simulink model "SIM_Patria_Microgrid"  (R2020b)
settings: Solver=ode23tb  StartTime=0.0  StopTime=24*60*60  FixedStep=1/(1000)  MaxStep=60  RelTol=1e-4
PreLoadFcn:
  | run('sim_initial_values.m')
StartFcn:
  | open_system('SIM_Patria_Microgrid/Scopes/ScopeSPS')
values from neighbouring files (symbols this model uses):
  data = get_scenario(1)    [sim_initial_values.m]
undefined symbols (not defined in the file or in its folder): Angle, Magnitude, params
libraries: powerlib x34, simulink x4
settings Model: ModifiedByFormat=SPS  ExtModeTrigMode=oneshot  ExtModeArmWhenConnect=off  Creator=MathWorks  LastModifiedBy=SPS
settings SolverCC: InitialStep=1e-4  ZeroCrossAlgorithm=Adaptive
settings DataIOCC: SaveFormat=Array  SignalLoggingSaveFormat=ModelDataLogs  SaveOutput=off  SaveTime=off  ReturnWorkspaceOutputs=off  SignalLoggingName=sigsOut
settings OptimizationCC: BooleanDataType=off  ExpressionDepthLimit=2147483647  InitFltsAndDblsToZero=on  LifeSpan=inf
settings DebuggingCC: AlgebraicLoopMsg=none  SaveWithParameterizedLinksMsg=none  UnderspecifiedInitializationDetection=Classic  MergeDetectMultiDrivingBlocksExec=none  SignalResolutionControl=TryResolveAllWithWarning  MultiTaskDSMMsg=warning  MultiTaskCondExecSysMsg=none  FcnCallInpInsideContextMsg=warning  AllowSymbolicDim=off  StateNameClashWarn=warning  SFUnexpectedBacktrackingDiag=warning  SFNoUnconditionalDefaultTransitionDiag=warning  SFExecutionAtInitializationDiag=none  ArithmeticOperatorsInVariantConditions=warning
settings HardwareCC: ProdBitPerPointer=32  ProdBitPerSizeT=32  ProdBitPerPtrDiffT=32  ProdLargestAtomicFloat=None  ProdIntDivRoundTo=Undefined  ProdEndianess=Unspecified  ProdWordSize=32  ProdHWDeviceType=32-bit Generic  TargetUnknown=on
settings ModelReferenceCC: PropagateSignalLabelsOutOfModel=off
settings SFSimCC: SimUseLocalCustomCode=off  CustomCodeUndefinedFunction=UseInterfaceOnly
settings RTWCC: RTWUseLocalCustomCode=off
settings CodeAppCC: StateflowObjectComments=on
settings GRTTargetCC: TargetFcnLib=ansi_tfl_tmw.mat  TargetLangStandard=C89/C90 (ANSI)  CombineOutputUpdateFcns=off  GRTInterface=on
settings ConfigComp: CovMetricSettings=dw  CovSaveCumulativeToWorkspaceVar=on  CovSaveSingleToWorkspaceVar=on  CovExternalEMLEnable=off  CovSFcnEnable=off
settings SimscapeCC: SimscapeNormalizeSystem=off

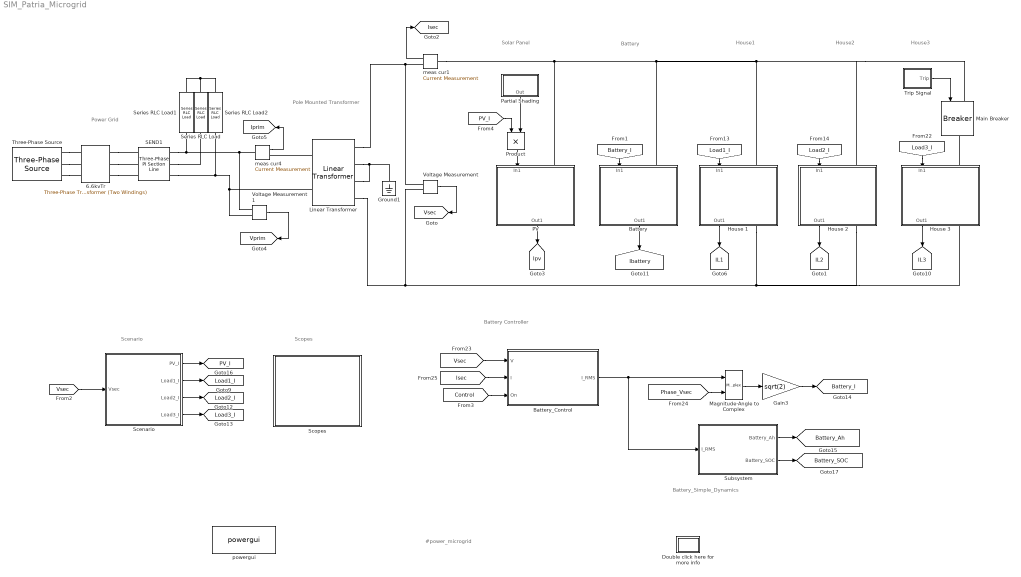
== system SIM_Patria_Microgrid ==
  note: Power Grid
  note: Pole Mounted
      | Transformer
  note: Solar Panel
  note: Battery
  note: House1
  note: House2
  note: House3
  note: Battery_Simple_Dynamics
  note: Battery Controller
  note: Scenario
  note: Scopes
  note: #power_microgrid
  6.6kvTr : powerlib/Elements/Three-Phase Transformer (Two Windings)  Winding1Connection=Yg  Winding2Connection=Y  CoreType=Three single-phase transformers  SetSaturation=off  Hysteresis=off  DataFile='hysteresis'  SetInitialFlux=off  Measurements=None  UNITS=pu  NominalPower=[ 10e6 , 60 ]  Winding1=[ 66e3 , 0.002 , 0.08 ]  Winding2=[6.6e3 , 0.002 , 0.08 ]  Rm=500  Lm=500  L0=0.5  Saturation=[ 0,0 ; 0.0024,1.2 ; 1.0,1.52 ]  InitialFluxes=[ 0.8 , -0.8 , 0.7 ]  BreakLoop=on  DiscreteSolver=Trapezoidal iterative  DataType=off  TransfoNumber=1
  Battery : Subsystem
      mask Display: image(imread(fullfile(matlabroot,'toolbox/physmod/powersys/DR/DRdemo/Battery.jpg')))
  Battery_Control : Subsystem
  Double click here for more info : Subsystem
      settings: OpenFcn=showdemo(bdroot(gcb))
      mask Display: disp('?')
  Gain3 : Gain  Gain=sqrt(2)
  Ground1 : powerlib/Elements/Ground  LConnTagsString=a
  House 1 : Subsystem
      mask Display: image(imread('house.jpg'))
  House 2 : Subsystem
      mask Display: image(imread('house.jpg'))
  House 3 : Subsystem
      mask Display: image(imread('house.jpg'))
  Linear Transformer : powerlib/Elements/Linear Transformer  UNITS=pu  NominalPower=[75e3 60]  winding1=[ 6600 0.00005 0.0002 ]  winding2=[ 100 0.00005 0.0002 ]  ThreeWindings=on  winding3=[ 100 0.00005 0.0002 ]  RmLm=[ 50 50 ]  Measurements=None  DataType=off
  Magnitude-Angle to Complex : MagnitudeAngleToComplex
  Main Breaker : powerlib/Elements/Breaker  InitialState=1  SwitchingTimes=[0 10 ]+8*3600  External=on  BreakerResistance=0.001  SnubberResistance=1e6  SnubberCapacitance=inf  Measurements=None  MoreParameters=off  NoBreakLoop=off
  PV : Subsystem
      mask Display: image(imread('pv.jpg'))
  Partial Shading : Subsystem  mask(Signal Disturbance){Hour=11, Minute=0, Second=0, Duration=20, Factor=0.3}
      mask prompts: Duration "Duration (s):"
      mask help: Within the specified time range defined by Start and Duration parameters, output is set to 'Factor'. Outside the specified time range output is kept at 1.0.
      mask init:
      | T2=(Hour-1)*60*60;    % Hour in seconds
      | T3=(Minute-1)*60;  % Minute in seconds
      | Ton=T2+T3+(Second-1);    % Beginning of fault (s)
      | Toff=Ton+Duration; % End of fault (s)
      mask TypeOptions Hour: 0 |      1 |      2 |      3 |      4 |      5 |      6 |      7 |      8 |      9 |     10 |     11 |     12 |     13 |     14 |     15 |     16 |     17 |     18 |     19 |     20 |     21 |     22 |     23
      mask TypeOptions Minute: 0 |      1 |      2 |      3 |      4 |      5 |      6 |      7 |      8 |      9 |     10 |     11 |     12 |     13 |     14 |     15 |     16 |     17 |     18 |     19 |     20 |     21 |     22 |     23 |     24 |     25 |     26 |     27 |     28 |     29 |     30 |     31 |     32 |     33 |     34 |     35 |     36 |     37 |     38 |     39 |     40 |     41 |     42 |     43 |     44 |     45 |     46 |     47 |     48 |     49 |     50 |     51 |     52 |     53 |     54 |     55 |     56 |     57 |     58 |     59
      mask TypeOptions Second: 0 |      1 |      2 |      3 |      4 |      5 |      6 |      7 |      8 |      9 |     10 |     11 |     12 |     13 |     14 |     15 |     16 |     17 |     18 |     19 |     20 |     21 |     22 |     23 |     24 |     25 |     26 |     27 |     28 |     29 |     30 |     31 |     32 |     33 |     34 |     35 |     36 |     37 |     38 |     39 |     40 |     41 |     42 |     43 |     44 |     45 |     46 |     47 |     48 |     49 |     50 |     51 |     52 |     53 |     54 |     55 |     56 |     57 |     58 |     59
      mask DialogControl Control2 Prompt: Start:
  Product : Product
  SEND1 : powerlib/Elements/Three-Phase PI Section Line  LConnTagsString=a|b|c  RConnTagsString=A|B|C  Length=1  Frequency=50  Resistances=[ 0.01273 0.3864]  Inductances="[ 0.9337e-3  4.1264e-3]"  Capacitances=[12.74e-9 7.751e-9]
  Scenario : Subsystem
  Scopes : Subsystem
  Series RLC Load : powerlib/Elements/Series RLC Load  LConnTagsString=a  RConnTagsString=__new0  NominalVoltage=1000  NominalFrequency=50  ActivePower=10e3  InductivePower=100  CapacitivePower=100  Setx0=off  InitialVoltage=0  SetiL0=off  InitialCurrent=0  Measurements=None  LoadType=constant Z
  Series RLC Load1 : powerlib/Elements/Series RLC Load  LConnTagsString=a  RConnTagsString=__new0  NominalVoltage=1000  NominalFrequency=50  ActivePower=100e3  InductivePower=100  CapacitivePower=100  Setx0=off  InitialVoltage=0  SetiL0=off  InitialCurrent=0  Measurements=None  LoadType=constant Z
  Series RLC Load2 : powerlib/Elements/Series RLC Load  LConnTagsString=a  RConnTagsString=__new0  NominalVoltage=1000  NominalFrequency=50  ActivePower=10e3  InductivePower=100  CapacitivePower=100  Setx0=off  InitialVoltage=0  SetiL0=off  InitialCurrent=0  Measurements=None  LoadType=constant Z
  Subsystem : Subsystem  mask{AH=5000}
      mask prompts: AH "Capacity[Ah]"
      mask Display: image(imread(fullfile(matlabroot,'toolbox/physmod/powersys/DR/DRdemo/Battery.jpg')))
  Three-Phase Source : powerlib/Electrical Sources/Three-Phase Source  InternalConnection=Yg  VoltagePhases=off  Voltage=66e3  PhaseAngle=0  Voltage_phases=[25e3 25e3 25e3]/sqrt(3)  PhaseAngles_phases=[0 -120 +120]  Frequency=params.network.frequency  NonIdealSource=on  SpecifyImpedance=on  Resistance=0.8929  Inductance=16.58e-3  ShortCircuitLevel=100e6  BaseVoltage=25e3  XRratio=7  BusType=swing  Pref=0  Qref=0  Prefabc=[10e3, 10e3, 10e3]  Qrefabc=[0, 0, 0]  Qmin=-inf  Qmax=inf
  Trip Signal : Subsystem  mask(Trip Signal for House Main Breaker){Hour=8, Minute=0, Second=0, FaultDuration=0}
      mask prompts: FaultDuration "Fault duration (s):"
      mask init:
      | T2=(Hour-1)*60*60;    % Hour in seconds
      | T3=(Minute-1)*60;  % Minute in seconds
      | Ton=T2+T3+(Second-1);    % Beginning of fault (s)
      | Toff=Ton+FaultDuration; % End of fault (s)
      mask TypeOptions Hour: 0 |      1 |      2 |      3 |      4 |      5 |      6 |      7 |      8 |      9 |     10 |     11 |     12 |     13 |     14 |     15 |     16 |     17 |     18 |     19 |     20 |     21 |     22 |     23
      mask TypeOptions Minute: 0 |      1 |      2 |      3 |      4 |      5 |      6 |      7 |      8 |      9 |     10 |     11 |     12 |     13 |     14 |     15 |     16 |     17 |     18 |     19 |     20 |     21 |     22 |     23 |     24 |     25 |     26 |     27 |     28 |     29 |     30 |     31 |     32 |     33 |     34 |     35 |     36 |     37 |     38 |     39 |     40 |     41 |     42 |     43 |     44 |     45 |     46 |     47 |     48 |     49 |     50 |     51 |     52 |     53 |     54 |     55 |     56 |     57 |     58 |     59
      mask TypeOptions Second: 0 |      1 |      2 |      3 |      4 |      5 |      6 |      7 |      8 |      9 |     10 |     11 |     12 |     13 |     14 |     15 |     16 |     17 |     18 |     19 |     20 |     21 |     22 |     23 |     24 |     25 |     26 |     27 |     28 |     29 |     30 |     31 |     32 |     33 |     34 |     35 |     36 |     37 |     38 |     39 |     40 |     41 |     42 |     43 |     44 |     45 |     46 |     47 |     48 |     49 |     50 |     51 |     52 |     53 |     54 |     55 |     56 |     57 |     58 |     59
      mask DialogControl Control2 Prompt: Fault timing:
  Voltage Measurement : powerlib/Measurements/Voltage Measurement  PhasorSimulation=on  OutputType=Complex  PSBequivalent=0
  Voltage Measurement1 : powerlib/Measurements/Voltage Measurement  PhasorSimulation=on  OutputType=Magnitude-Angle  PSBequivalent=0
  meas cur1 : powerlib/Measurements/Current Measurement  PhasorSimulation=on  OutputType=Complex  PSBequivalent=0
  meas cur4 : powerlib/Measurements/Current Measurement  PhasorSimulation=on  OutputType=Magnitude-Angle  PSBequivalent=0
  powergui : powerlib/powergui  SimulationMode=Phasor  SampleTime=1/60/100  frequency=50  Iterations=50  frequencyindice=60  Pbase=100e6  ErrMax=1e-4  UnitsV=kV  UnitsW=MW  buscounter=0  FunctionMessages=off  echomessages=off  EnableUseOfTLC=off  CurrentSourceSwitches=off  DisableSnubberDevices=off  DisableRonSwitches=off  DisableVfSwitches=off  DisplayEquations=off  AutomaticDiscreteSolvers=off  SolverType=Tustin  Interpol=off  ExternalGateDelay=off  methode=off  Ts=0  x0status=blocks  SPID=off  SwTol=0  HookPort=off  NonlinearTolerance=0  nMaxIteration=15  ContinueOnMaxIteration=off  RestoreLinks=warning  ResistiveCurrentMeasurement=off  Frange=[0:2:500]  Ylog=off  Xlog=on  ShowGrid=off  save=off  variable=ZData  structure=0  ZoomFFT=on  StartTime=0.0  cycles=1  DisplayStyle=1  fundamental=60  FreqAxis=off  MaxFrequency=1000  frequencyindicesteady=1  RmsSteady=1  display=off
  tag scope: Battery_Ah=global, Battery_I=global, Battery_SOC=global, IL1=global, IL2=global, IL3=global, Ibattery=global, Iprim=global, Ipv=global, Isec=global, Load1_I=global, Load2_I=global, Load3_I=global, PV_I=global, Vprim=global, Vsec=global
  wires:
  House 2/1(Out1) -> [IL2]
  House 1/1(Out1) -> [IL1]
  meas cur1/1 -> [Isec]
  House 3/1(Out1) -> [IL3]
  [Load2_I] -> House 2/1(In1)
  [Load3_I] -> House 3/1(In1)
  [Battery_I] -> Battery/1(In1)
  Subsystem/1(Battery_Ah) -> [Battery_Ah]
  Subsystem/2(Battery_SOC) -> [Battery_SOC]
  PV/1(Out1) -> [Ipv]
  Battery/1(Out1) -> [Ibattery]
  [Phase_Vsec] -> Magnitude-Angle to Complex/2
  Magnitude-Angle to Complex/1 -> Gain3/1
  Gain3/1 -> [Battery_I]
  Battery_Control/1(I_RMS) -> Magnitude-Angle to Complex/1, Subsystem/1(I_RMS)
  Scenario/1(PV_I) -> [PV_I]
  Scenario/2(Load1_I) -> [Load1_I]
  Scenario/3(Load2_I) -> [Load2_I]
  Scenario/4(Load3_I) -> [Load3_I]
  [Vsec] -> Scenario/1(Vsec)
  Voltage Measurement1/1 -> [Vprim]
  meas cur4/1 -> [Iprim]
  [Load1_I] -> House 1/1(In1)
  Voltage Measurement/1 -> [Vsec]
  [Isec] -> Battery_Control/2(I)
  [Vsec] -> Battery_Control/1(V)
  [Control] -> Battery_Control/3(On)
  Trip Signal/1(Trip) -> Main Breaker/1
  [PV_I] -> Product/1
  Product/1 -> PV/1(In1)
  Partial Shading/1(Out) -> Product/2
  connections:
  SEND1/RConn1 -- meas cur4/LConn1 -- Voltage Measurement1/LConn1 -- Series RLC Load1/RConn1
  SEND1/RConn3 -- Linear Transformer/LConn2 -- Voltage Measurement1/LConn2 -- Series RLC Load2/RConn1
  6.6kvTr/RConn2 -- SEND1/LConn2
  6.6kvTr/RConn1 -- SEND1/LConn1
  Three-Phase Source/RConn1 -- 6.6kvTr/LConn1
  Three-Phase Source/RConn3 -- 6.6kvTr/LConn3
  6.6kvTr/RConn3 -- SEND1/LConn3
  Ground1/LConn1 -- Linear Transformer/RConn3 -- Linear Transformer/RConn2
  Three-Phase Source/RConn2 -- 6.6kvTr/LConn2
  SEND1/RConn2 -- Series RLC Load/RConn1
  Series RLC Load1/LConn1 -- Series RLC Load/LConn1 -- Series RLC Load2/LConn1
  Linear Transformer/LConn1 -- meas cur4/RConn1
  Voltage Measurement/LConn1 -- Linear Transformer/RConn1 -- meas cur1/RConn1
  Voltage Measurement/LConn2 -- Linear Transformer/RConn4 -- House 2/RConn1 -- House 3/RConn1 -- House 1/RConn1
  meas cur1/LConn1 -- House 1/LConn1 -- Main Breaker/LConn1 -- House 2/LConn1 -- Battery/LConn1 -- PV/LConn1
  House 3/LConn1 -- Main Breaker/RConn1

== system SIM_Patria_Microgrid/Battery ==
  In1 : Inport
  Controlled Current Source1 : powerlib/Electrical Sources/Controlled Current Source  Initialize=on  Source_Type=AC  Amplitude=0  Phase=30  Frequency=60  Measurements=None
  Ground3 : powerlib/Elements/Ground  LConnTagsString=a
  Snubber : powerlib/Elements/Series RLC Branch  LConnTagsString=__new0  RConnTagsString=__new0  BranchType=R  Resistance=1e6  Inductance=1e-3  SetiL0=off  InitialCurrent=0  Capacitance=1e-6  Setx0=off  InitialVoltage=0  Measurements=None
  meas cur6 : powerlib/Measurements/Current Measurement  PhasorSimulation=on  OutputType=Complex  PSBequivalent=0
  Conn1 : PMIOPort  Side=Left
  Out1 : Outport  VectorParamsAs1DForOutWhenUnconnected=off
  wires:
  meas cur6/1 -> Out1/1
  In1/1 -> Controlled Current Source1/1
  connections:
  Controlled Current Source1/LConn1 -- Ground3/LConn1 -- Snubber/RConn1
  Controlled Current Source1/RConn1 -- Snubber/LConn1 -- meas cur6/LConn1
  Conn1/RConn1 -- meas cur6/RConn1

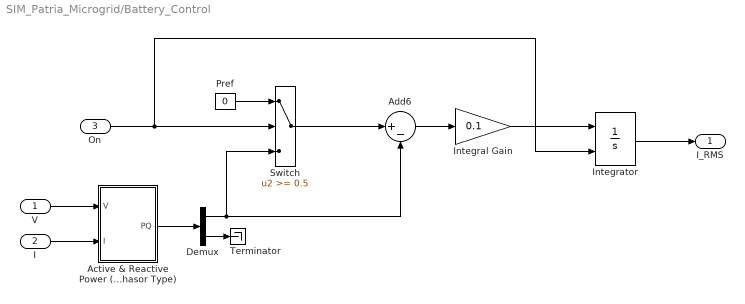
== system SIM_Patria_Microgrid/Battery_Control ==
  V : Inport
  I : Inport  Port=2
  On : Inport  Port=3
  Active & Reactive Power (Phasor Type) : Subsystem  DialogController=POWERSYS.PowerSysDialog  mask(Active & Reactive Power (Phasor Type)){}
      mask help: Active & Reactive Power (Phasor Type)
      mask init:
      | power_initmask();
      mask Help: This block is part of a subset of blocks in the Extras library that does not have documentation associated with it, other than the block mask description.
      mask Display: disp('')
  Add6 : Sum  Inputs=|+-
  Demux : Demux  Outputs=2
  Integral Gain : Gain  Gain=0.1
  Integrator : Integrator  ExternalReset=falling  LimitOutput=on  UpperSaturationLimit=50  LowerSaturationLimit=-50
  Pref : Constant  Value=0
  Switch : Switch  Threshold=0.5
  Terminator : Terminator
  I_RMS : Outport  OutputWhenDisabled=reset  InitialOutput=0  VectorParamsAs1DForOutWhenUnconnected=off
  wires:
  Pref/1 -> Switch/1
  Integrator/1 -> I_RMS/1
  On/1 -> Integrator/2, Switch/2
  Add6/1 -> Integral Gain/1
  Integral Gain/1 -> Integrator/1
  Demux/1 -> Switch/3, Add6/2
  Active & Reactive Power (Phasor Type)/1(PQ) -> Demux/1
  I/1 -> Active & Reactive Power (Phasor Type)/2(I)
  V/1 -> Active & Reactive Power (Phasor Type)/1(V)
  Demux/2 -> Terminator/1
  Switch/1 -> Add6/1

== system SIM_Patria_Microgrid/Double click here for more info ==

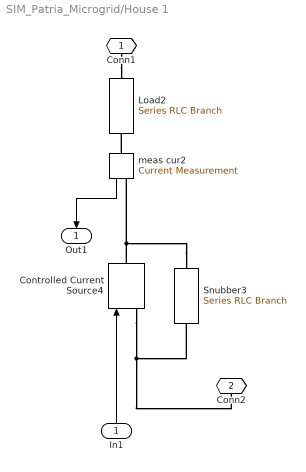
== system SIM_Patria_Microgrid/House 1 ==
  In1 : Inport
  Controlled Current Source4 : powerlib/Electrical Sources/Controlled Current Source  Initialize=on  Source_Type=AC  Amplitude=0  Phase=30  Frequency=60  Measurements=None
  Load2 : powerlib/Elements/Series RLC Branch  LConnTagsString=__new0  RConnTagsString=__new0  BranchType=R  Resistance=16  Inductance=1e-3  SetiL0=off  InitialCurrent=0  Capacitance=1e-6  Setx0=off  InitialVoltage=0  Measurements=None
  Snubber3 : powerlib/Elements/Series RLC Branch  LConnTagsString=__new0  RConnTagsString=__new0  BranchType=R  Resistance=1e6  Inductance=1e-3  SetiL0=off  InitialCurrent=0  Capacitance=1e-6  Setx0=off  InitialVoltage=0  Measurements=None
  meas cur2 : powerlib/Measurements/Current Measurement  PhasorSimulation=on  OutputType=Complex  PSBequivalent=0
  Conn1 : PMIOPort  Side=Left
  Conn2 : PMIOPort  Port=2  Side=Right
  Out1 : Outport  VectorParamsAs1DForOutWhenUnconnected=off
  wires:
  In1/1 -> Controlled Current Source4/1
  meas cur2/1 -> Out1/1
  connections:
  Conn1/RConn1 -- Load2/LConn1
  meas cur2/LConn1 -- Load2/RConn1
  Snubber3/LConn1 -- meas cur2/RConn1 -- Controlled Current Source4/RConn1
  Snubber3/RConn1 -- Conn2/RConn1 -- Controlled Current Source4/LConn1

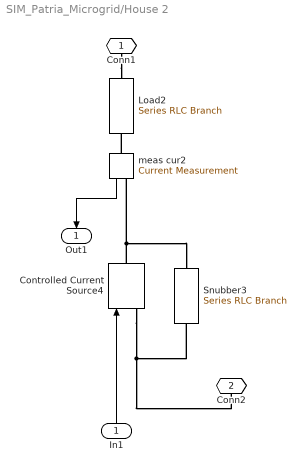
== system SIM_Patria_Microgrid/House 2 ==
  In1 : Inport
  Controlled Current Source4 : powerlib/Electrical Sources/Controlled Current Source  Initialize=on  Source_Type=AC  Amplitude=0  Phase=30  Frequency=60  Measurements=None
  Load2 : powerlib/Elements/Series RLC Branch  LConnTagsString=__new0  RConnTagsString=__new0  BranchType=R  Resistance=16  Inductance=1e-3  SetiL0=off  InitialCurrent=0  Capacitance=1e-6  Setx0=off  InitialVoltage=0  Measurements=None
  Snubber3 : powerlib/Elements/Series RLC Branch  LConnTagsString=__new0  RConnTagsString=__new0  BranchType=R  Resistance=1e6  Inductance=1e-3  SetiL0=off  InitialCurrent=0  Capacitance=1e-6  Setx0=off  InitialVoltage=0  Measurements=None
  meas cur2 : powerlib/Measurements/Current Measurement  PhasorSimulation=on  OutputType=Complex  PSBequivalent=0
  Conn1 : PMIOPort  Side=Left
  Conn2 : PMIOPort  Port=2  Side=Right
  Out1 : Outport  VectorParamsAs1DForOutWhenUnconnected=off
  wires:
  meas cur2/1 -> Out1/1
  In1/1 -> Controlled Current Source4/1
  connections:
  Controlled Current Source4/LConn1 -- Conn2/RConn1 -- Snubber3/RConn1
  Controlled Current Source4/RConn1 -- meas cur2/RConn1 -- Snubber3/LConn1
  meas cur2/LConn1 -- Load2/RConn1
  Conn1/RConn1 -- Load2/LConn1

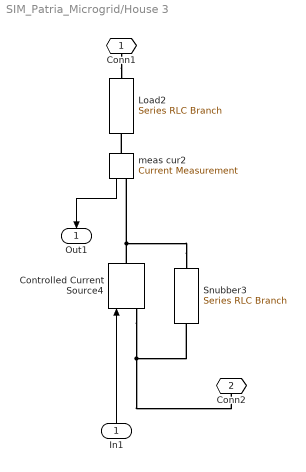
== system SIM_Patria_Microgrid/House 3 ==
  In1 : Inport
  Controlled Current Source4 : powerlib/Electrical Sources/Controlled Current Source  Initialize=on  Source_Type=AC  Amplitude=0  Phase=30  Frequency=60  Measurements=None
  Load2 : powerlib/Elements/Series RLC Branch  LConnTagsString=__new0  RConnTagsString=__new0  BranchType=R  Resistance=16  Inductance=1e-3  SetiL0=off  InitialCurrent=0  Capacitance=1e-6  Setx0=off  InitialVoltage=0  Measurements=None
  Snubber3 : powerlib/Elements/Series RLC Branch  LConnTagsString=__new0  RConnTagsString=__new0  BranchType=R  Resistance=1e6  Inductance=1e-3  SetiL0=off  InitialCurrent=0  Capacitance=1e-6  Setx0=off  InitialVoltage=0  Measurements=None
  meas cur2 : powerlib/Measurements/Current Measurement  PhasorSimulation=on  OutputType=Complex  PSBequivalent=0
  Conn1 : PMIOPort  Side=Left
  Conn2 : PMIOPort  Port=2  Side=Right
  Out1 : Outport  VectorParamsAs1DForOutWhenUnconnected=off
  wires:
  In1/1 -> Controlled Current Source4/1
  meas cur2/1 -> Out1/1
  connections:
  Conn1/RConn1 -- Load2/LConn1
  meas cur2/LConn1 -- Load2/RConn1
  Snubber3/LConn1 -- meas cur2/RConn1 -- Controlled Current Source4/RConn1
  Snubber3/RConn1 -- Conn2/RConn1 -- Controlled Current Source4/LConn1

== system SIM_Patria_Microgrid/PV ==
  In1 : Inport
  Controlled Current Source : powerlib/Electrical Sources/Controlled Current Source  Initialize=on  Source_Type=AC  Amplitude=0  Phase=30  Frequency=60  Measurements=None
  Ground2 : powerlib/Elements/Ground  LConnTagsString=a
  Snubber1 : powerlib/Elements/Series RLC Branch  LConnTagsString=__new0  RConnTagsString=__new0  BranchType=R  Resistance=1e6  Inductance=1e-3  SetiL0=off  InitialCurrent=0  Capacitance=1e-6  Setx0=off  InitialVoltage=0  Measurements=None
  meas cur3 : powerlib/Measurements/Current Measurement  PhasorSimulation=on  OutputType=Complex  PSBequivalent=0
  Conn1 : PMIOPort  Side=Left
  Out1 : Outport  VectorParamsAs1DForOutWhenUnconnected=off
  wires:
  meas cur3/1 -> Out1/1
  In1/1 -> Controlled Current Source/1
  connections:
  Ground2/LConn1 -- Controlled Current Source/LConn1 -- Snubber1/RConn1
  Snubber1/LConn1 -- Controlled Current Source/RConn1 -- meas cur3/LConn1
  Conn1/RConn1 -- meas cur3/RConn1

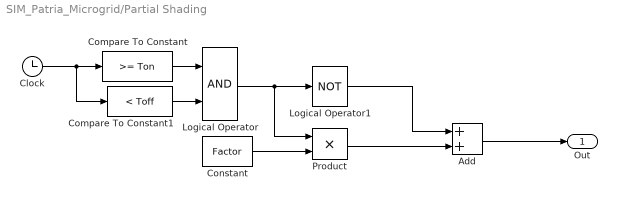
== system SIM_Patria_Microgrid/Partial Shading ==
  Add : Sum
  Clock : Clock
  Compare To Constant : simulink/Logic and Bit Operations/Compare To Constant  relop=>=  const=Ton  OutDataTypeStr=boolean
  Compare To Constant1 : simulink/Logic and Bit Operations/Compare To Constant  relop=<  const=Toff  OutDataTypeStr=boolean
  Constant : Constant  Value=Factor
  Logical Operator : Logic  AllPortsSameDT=off  OutDataTypeStr=float('double')
  Logical Operator1 : Logic  Operator=NOT  AllPortsSameDT=off  OutDataTypeStr=float('double')
  Product : Product
  Out : Outport  VectorParamsAs1DForOutWhenUnconnected=off
  wires:
  Add/1 -> Out/1
  Product/1 -> Add/2
  Constant/1 -> Product/2
  Compare To Constant/1 -> Logical Operator/1
  Clock/1 -> Compare To Constant1/1, Compare To Constant/1
  Compare To Constant1/1 -> Logical Operator/2
  Logical Operator/1 -> Logical Operator1/1, Product/1
  Logical Operator1/1 -> Add/1

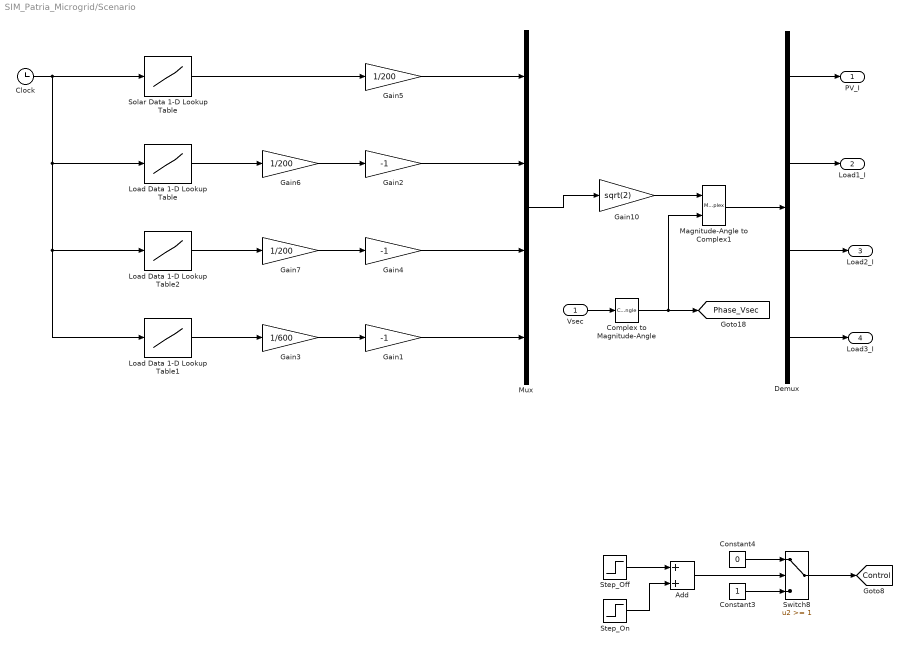
== system SIM_Patria_Microgrid/Scenario ==
  Vsec : Inport
  Add : Sum
  Clock : Clock
  Complex to Magnitude-Angle : ComplexToMagnitudeAngle  Output=Angle
  Constant3 : Constant
  Constant4 : Constant  Value=0
  Demux : Demux
  Gain1 : Gain  Gain=-1
  Gain10 : Gain  Gain=sqrt(2)
  Gain2 : Gain  Gain=-1
  Gain3 : Gain  Gain=1/600
  Gain4 : Gain  Gain=-1
  Gain5 : Gain  Gain=1/200
  Gain6 : Gain  Gain=1/200
  Gain7 : Gain  Gain=1/200
  Load Data 1-D Lookup Table : Lookup_n-D  NumberOfTableDimensions=1  BreakpointsForDimension1=data.time  BeginIndexSearchUsingPreviousIndexResult=on  Table=data.P11min  InternalRulePriority=Speed  RndMeth=Simplest  InputSameDT=on
  Load Data 1-D Lookup Table1 : Lookup_n-D  NumberOfTableDimensions=1  BreakpointsForDimension1=data.time  BeginIndexSearchUsingPreviousIndexResult=on  Table=data.P31min  InternalRulePriority=Speed  RndMeth=Simplest  InputSameDT=on
  Load Data 1-D Lookup Table2 : Lookup_n-D  NumberOfTableDimensions=1  BreakpointsForDimension1=data.time  BeginIndexSearchUsingPreviousIndexResult=on  Table=data.P21min  InternalRulePriority=Speed  RndMeth=Simplest  InputSameDT=on
  Magnitude-Angle to Complex1 : MagnitudeAngleToComplex
  Mux : Mux
  Solar Data 1-D Lookup Table : Lookup_n-D  NumberOfTableDimensions=1  BreakpointsForDimension1=params.solar.SPT_1min  BeginIndexSearchUsingPreviousIndexResult=on  Table=params.solar.SPD_1min  InternalRulePriority=Speed  RndMeth=Simplest  InputSameDT=on
  Step_Off : Step  Time=1*60*60  SampleTime=0
  Step_On : Step  Time=6*60*60  After=-1  SampleTime=0
  Switch8 : Switch  Threshold=1
  PV_I : Outport  VectorParamsAs1DForOutWhenUnconnected=off
  Load1_I : Outport  Port=2  VectorParamsAs1DForOutWhenUnconnected=off
  Load2_I : Outport  Port=3  VectorParamsAs1DForOutWhenUnconnected=off
  Load3_I : Outport  Port=4  VectorParamsAs1DForOutWhenUnconnected=off
  tag scope: Control=global, Phase_Vsec=global
  wires:
  Switch8/1 -> [Control]
  Constant4/1 -> Switch8/1
  Gain6/1 -> Gain2/1
  Mux/1 -> Gain10/1
  Gain10/1 -> Magnitude-Angle to Complex1/1
  Magnitude-Angle to Complex1/1 -> Demux/1
  Demux/1 -> PV_I/1
  Gain5/1 -> Mux/1
  Constant3/1 -> Switch8/3
  Vsec/1 -> Complex to Magnitude-Angle/1
  Complex to Magnitude-Angle/1 -> Magnitude-Angle to Complex1/2, [Phase_Vsec]
  Step_Off/1 -> Add/1
  Step_On/1 -> Add/2
  Add/1 -> Switch8/2
  Solar Data 1-D Lookup Table/1 -> Gain5/1
  Load Data 1-D Lookup Table/1 -> Gain6/1
  Gain3/1 -> Gain1/1
  Load Data 1-D Lookup Table1/1 -> Gain3/1
  Clock/1 -> Load Data 1-D Lookup Table/1, Load Data 1-D Lookup Table1/1, Load Data 1-D Lookup Table2/1, Solar Data 1-D Lookup Table/1
  Gain7/1 -> Gain4/1
  Load Data 1-D Lookup Table2/1 -> Gain7/1
  Gain2/1 -> Mux/2
  Gain4/1 -> Mux/3
  Gain1/1 -> Mux/4
  Demux/2 -> Load1_I/1
  Demux/3 -> Load2_I/1
  Demux/4 -> Load3_I/1

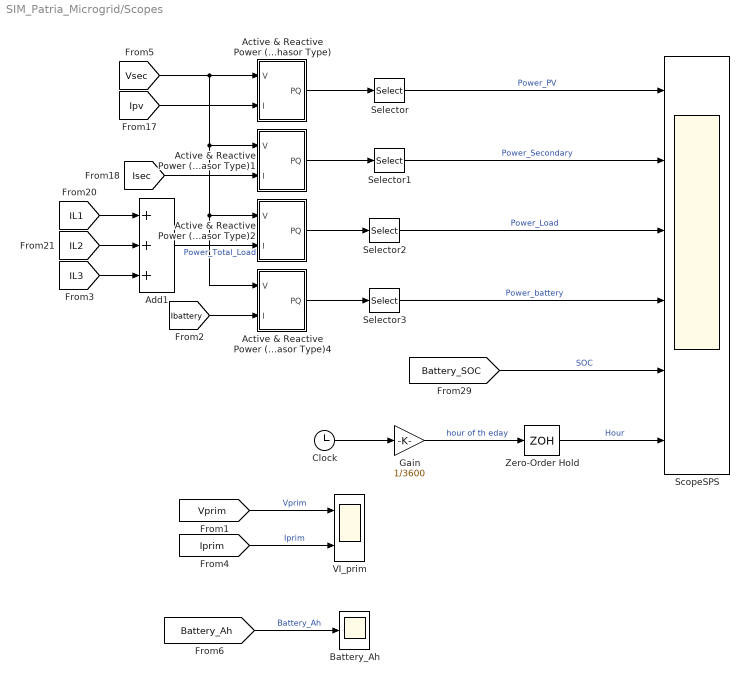
== system SIM_Patria_Microgrid/Scopes ==
  Active & Reactive Power (Phasor Type) : Subsystem  DialogController=POWERSYS.PowerSysDialog  mask(Active & Reactive Power (Phasor Type)){}
      mask help: Active & Reactive Power (Phasor Type)
      mask init:
      | power_initmask();
      mask Help: This block is part of a subset of blocks in the Extras library that does not have documentation associated with it, other than the block mask description.
      mask Display: disp('')
  Active & Reactive Power (Phasor Type)1 : Subsystem  DialogController=POWERSYS.PowerSysDialog  mask(Active & Reactive Power (Phasor Type)){}
      mask help: Active & Reactive Power (Phasor Type)
      mask init:
      | power_initmask();
      mask Help: This block is part of a subset of blocks in the Extras library that does not have documentation associated with it, other than the block mask description.
      mask Display: disp('')
  Active & Reactive Power (Phasor Type)2 : Subsystem  DialogController=POWERSYS.PowerSysDialog  mask(Active & Reactive Power (Phasor Type)){}
      mask help: Active & Reactive Power (Phasor Type)
      mask init:
      | power_initmask();
      mask Help: This block is part of a subset of blocks in the Extras library that does not have documentation associated with it, other than the block mask description.
      mask Display: disp('')
  Active & Reactive Power (Phasor Type)4 : Subsystem  DialogController=POWERSYS.PowerSysDialog  mask(Active & Reactive Power (Phasor Type)){}
      mask help: Active & Reactive Power (Phasor Type)
      mask init:
      | power_initmask();
      mask Help: This block is part of a subset of blocks in the Extras library that does not have documentation associated with it, other than the block mask description.
      mask Display: disp('')
  Add1 : Sum  Inputs=+++
  Battery_Ah : Scope
  Clock : Clock
  Gain : Gain  Gain=1/3600
  ScopeSPS : Scope  NumInputPorts=6
  Selector{,1..3} (4 alike) : Selector  InputPortWidth=2  IndexOptions=Index vector (dialog)  Indices=1  OutputSizes=1
  VI_prim : Scope  NumInputPorts=2
  Zero-Order Hold : ZeroOrderHold  SampleTime=3600
  wires:
  [Ipv] -> Active & Reactive Power (Phasor Type)/2(I)
  [Vsec] -> Active & Reactive Power (Phasor Type)4/1(V), Active & Reactive Power (Phasor Type)2/1(V), Active & Reactive Power (Phasor Type)1/1(V), Active & Reactive Power (Phasor Type)/1(V)
  Active & Reactive Power (Phasor Type)/1(PQ) -> Selector/1
  Selector/1 -> ScopeSPS/1  "Power_PV"
  [IL1] -> Add1/1
  [IL2] -> Add1/2
  [IL3] -> Add1/3
  [Isec] -> Active & Reactive Power (Phasor Type)1/2(I)
  Add1/1 -> Active & Reactive Power (Phasor Type)2/2(I)  "Power_Total_Load"
  [Ibattery] -> Active & Reactive Power (Phasor Type)4/2(I)
  Active & Reactive Power (Phasor Type)1/1(PQ) -> Selector1/1
  Active & Reactive Power (Phasor Type)2/1(PQ) -> Selector2/1
  Active & Reactive Power (Phasor Type)4/1(PQ) -> Selector3/1
  Selector1/1 -> ScopeSPS/2  "Power_Secondary"
  Selector2/1 -> ScopeSPS/3  "Power_Load"
  Selector3/1 -> ScopeSPS/4  "Power_battery"
  [Battery_SOC] -> ScopeSPS/5  "SOC"
  [Vprim] -> VI_prim/1  "Vprim"
  [Iprim] -> VI_prim/2  "Iprim"
  [Battery_Ah] -> Battery_Ah/1  "Battery_Ah"
  Clock/1 -> Gain/1
  Gain/1 -> Zero-Order Hold/1  "hour of th eday"
  Zero-Order Hold/1 -> ScopeSPS/6  "Hour"

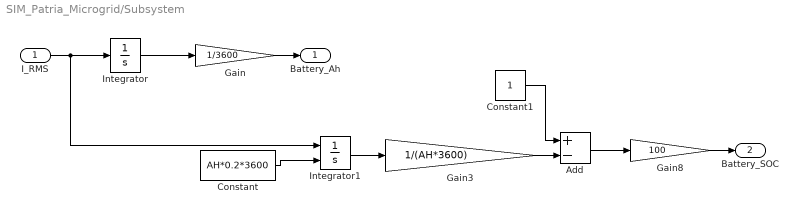
== system SIM_Patria_Microgrid/Subsystem ==
  I_RMS : Inport
  Add : Sum  Inputs=+-
  Constant : Constant  Value=AH*0.2*3600
  Constant1 : Constant
  Gain : Gain  Gain=1/3600
  Gain3 : Gain  Gain=1/(AH*3600)
  Gain8 : Gain  Gain=100
  Integrator : Integrator
  Integrator1 : Integrator  InitialConditionSource=external
  Battery_Ah : Outport  VectorParamsAs1DForOutWhenUnconnected=off
  Battery_SOC : Outport  Port=2  VectorParamsAs1DForOutWhenUnconnected=off
  wires:
  Integrator/1 -> Gain/1
  Integrator1/1 -> Gain3/1
  Gain3/1 -> Add/2
  Constant1/1 -> Add/1
  Add/1 -> Gain8/1
  Constant/1 -> Integrator1/2
  I_RMS/1 -> Integrator/1, Integrator1/1
  Gain/1 -> Battery_Ah/1
  Gain8/1 -> Battery_SOC/1

== system SIM_Patria_Microgrid/Trip Signal ==
  note: 0 = TRIP
  Clock : Clock
  Compare To Constant : simulink/Logic and Bit Operations/Compare To Constant  relop=>=  const=Ton  OutDataTypeStr=boolean
  Compare To Constant1 : simulink/Logic and Bit Operations/Compare To Constant  relop=<  const=Toff  OutDataTypeStr=boolean
  Logical Operator : Logic  AllPortsSameDT=off  OutDataTypeStr=float('double')
  Logical Operator1 : Logic  Operator=NOT  AllPortsSameDT=off  OutDataTypeStr=float('double')
  Trip : Outport  VectorParamsAs1DForOutWhenUnconnected=off
  wires:
  Compare To Constant/1 -> Logical Operator/1
  Clock/1 -> Compare To Constant1/1, Compare To Constant/1
  Compare To Constant1/1 -> Logical Operator/2
  Logical Operator/1 -> Logical Operator1/1
  Logical Operator1/1 -> Trip/1

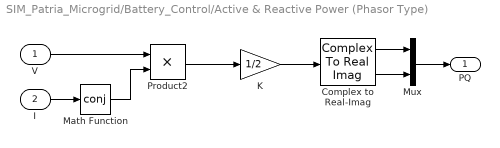
== system SIM_Patria_Microgrid/Battery_Control/Active & Reactive Power (Phasor Type) ==
  V : Inport
  I : Inport  Port=2
  Complex to Real-Imag : ComplexToRealImag
  K : Gain  Gain=1/2  SaturateOnIntegerOverflow=on  OutDataTypeStr=Inherit: Same as input  ParamDataTypeStr=Inherit: Same as input
  Math Function : Math  Operator=conj  SignedPower=on  SaturateOnIntegerOverflow=on
  Mux : Mux  Inputs=2
  Product2 : Product  InputSameDT=on  SaturateOnIntegerOverflow=on  OutDataTypeStr=Inherit: Same as first input
  PQ : Outport  VectorParamsAs1DForOutWhenUnconnected=off
  wires:
  Mux/1 -> PQ/1
  Complex to Real-Imag/2 -> Mux/2
  Complex to Real-Imag/1 -> Mux/1
  V/1 -> Product2/1
  Math Function/1 -> Product2/2
  Product2/1 -> K/1
  K/1 -> Complex to Real-Imag/1
  I/1 -> Math Function/1

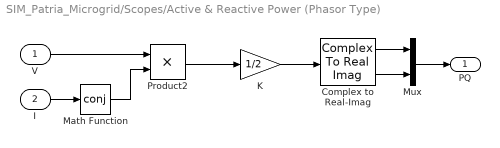
== system SIM_Patria_Microgrid/Scopes/Active & Reactive Power (Phasor Type) ==
  V : Inport
  I : Inport  Port=2
  Complex to Real-Imag : ComplexToRealImag
  K : Gain  Gain=1/2  SaturateOnIntegerOverflow=on  OutDataTypeStr=Inherit: Same as input  ParamDataTypeStr=Inherit: Same as input
  Math Function : Math  Operator=conj  SignedPower=on  SaturateOnIntegerOverflow=on
  Mux : Mux  Inputs=2
  Product2 : Product  InputSameDT=on  SaturateOnIntegerOverflow=on  OutDataTypeStr=Inherit: Same as first input
  PQ : Outport  VectorParamsAs1DForOutWhenUnconnected=off
  wires:
  Mux/1 -> PQ/1
  Complex to Real-Imag/2 -> Mux/2
  Complex to Real-Imag/1 -> Mux/1
  V/1 -> Product2/1
  Math Function/1 -> Product2/2
  Product2/1 -> K/1
  K/1 -> Complex to Real-Imag/1
  I/1 -> Math Function/1

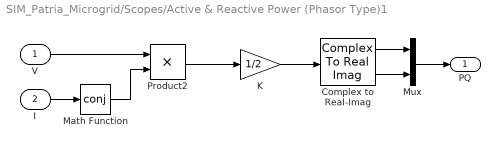
== system SIM_Patria_Microgrid/Scopes/Active & Reactive Power (Phasor Type)1 ==
  V : Inport
  I : Inport  Port=2
  Complex to Real-Imag : ComplexToRealImag
  K : Gain  Gain=1/2  SaturateOnIntegerOverflow=on  OutDataTypeStr=Inherit: Same as input  ParamDataTypeStr=Inherit: Same as input
  Math Function : Math  Operator=conj  SignedPower=on  SaturateOnIntegerOverflow=on
  Mux : Mux  Inputs=2
  Product2 : Product  InputSameDT=on  SaturateOnIntegerOverflow=on  OutDataTypeStr=Inherit: Same as first input
  PQ : Outport  VectorParamsAs1DForOutWhenUnconnected=off
  wires:
  Mux/1 -> PQ/1
  Complex to Real-Imag/2 -> Mux/2
  Complex to Real-Imag/1 -> Mux/1
  V/1 -> Product2/1
  Math Function/1 -> Product2/2
  Product2/1 -> K/1
  K/1 -> Complex to Real-Imag/1
  I/1 -> Math Function/1

== system SIM_Patria_Microgrid/Scopes/Active & Reactive Power (Phasor Type)2 ==
  V : Inport
  I : Inport  Port=2
  Complex to Real-Imag : ComplexToRealImag
  K : Gain  Gain=1/2  SaturateOnIntegerOverflow=on  OutDataTypeStr=Inherit: Same as input  ParamDataTypeStr=Inherit: Same as input
  Math Function : Math  Operator=conj  SignedPower=on  SaturateOnIntegerOverflow=on
  Mux : Mux  Inputs=2
  Product2 : Product  InputSameDT=on  SaturateOnIntegerOverflow=on  OutDataTypeStr=Inherit: Same as first input
  PQ : Outport  VectorParamsAs1DForOutWhenUnconnected=off
  wires:
  Mux/1 -> PQ/1
  Complex to Real-Imag/2 -> Mux/2
  Complex to Real-Imag/1 -> Mux/1
  V/1 -> Product2/1
  Math Function/1 -> Product2/2
  Product2/1 -> K/1
  K/1 -> Complex to Real-Imag/1
  I/1 -> Math Function/1

== system SIM_Patria_Microgrid/Scopes/Active & Reactive Power (Phasor Type)4 ==
  V : Inport
  I : Inport  Port=2
  Complex to Real-Imag : ComplexToRealImag
  K : Gain  Gain=1/2  SaturateOnIntegerOverflow=on  OutDataTypeStr=Inherit: Same as input  ParamDataTypeStr=Inherit: Same as input
  Math Function : Math  Operator=conj  SignedPower=on  SaturateOnIntegerOverflow=on
  Mux : Mux  Inputs=2
  Product2 : Product  InputSameDT=on  SaturateOnIntegerOverflow=on  OutDataTypeStr=Inherit: Same as first input
  PQ : Outport  VectorParamsAs1DForOutWhenUnconnected=off
  wires:
  Mux/1 -> PQ/1
  Complex to Real-Imag/2 -> Mux/2
  Complex to Real-Imag/1 -> Mux/1
  V/1 -> Product2/1
  Math Function/1 -> Product2/2
  Product2/1 -> K/1
  K/1 -> Complex to Real-Imag/1
  I/1 -> Math Function/1
